simulink model "simTC"  (R2015a)
settings: Solver=ode4  StartTime=0.0  StopTime=T_sim  FixedStep=Ts  RelTol=1e-3
values from neighbouring files (symbols this model uses):
  A = [A, B; zeros(nu, nu+nx)]    [Main.m]    (also in longitudinal_inputRate.mat = [-0.0720238415998 -0.037172929775 0 2.59473518947e-15 0 0 8.; longitudinal_mat.mat = [-0.0720238415998 -0.037172929775 0 2.59473518947e-15 8.2339)
  B = [zeros(nx, nu); eye(nu)]    [Main.m]    (also in longitudinal_inputRate.mat = [0  0; 0  0; 0  0; 0  0; 1  0; 0  1]; longitudinal_mat.mat = [-0.11942228308  27.1604492573; -0.362246328988  0.037187163)
  C = [0 0 1 0 0 0]    [Main.m]    (also in main_CG.m = eye(nx); main_TC.m; main_TD.m = eye(nx))
  K_fb = K(:,1:nx)    [Main.m]    (also in main_TC.m)
  K_ff = K(:,nx+1:end)    [Main.m]    (also in main_TC.m)
  nx = size(Phi,1)    [CG_Offline.m]
  ref = 10    [Main.m]    (also in main_TC.m; main_TD.m)
undefined symbols (not defined in the file or in its folder): nu
settings Model: CovSFcnEnable=off  Creator=pier  LastModifiedBy=Piero
settings DebuggingCC: SolverPrmCheckMsg=warning

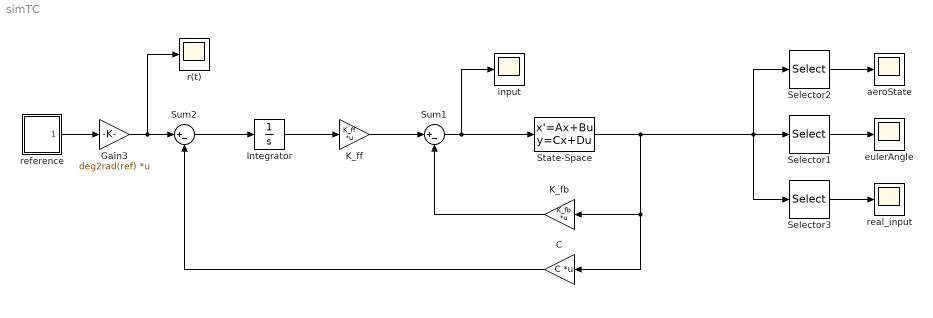
== system simTC ==
  C : Gain  Gain=C  Multiplication=Matrix(K*u)
  Gain3 : Gain  Gain=deg2rad(ref)  Multiplication=Matrix(K*u)
  Integrator : Integrator
  K_fb : Gain  Gain=K_fb  Multiplication=Matrix(K*u)
  K_ff : Gain  Gain=K_ff  Multiplication=Matrix(K*u)
  Selector1 : Selector  InputPortWidth=6  Indices=[3:4]
  Selector2 : Selector  InputPortWidth=6  Indices=[1:2]
  Selector3 : Selector  InputPortWidth=6  Indices=[5:6]
  State-Space : StateSpace  A=A  B=B  C=eye(nx)  D=zeros(nx,nu)  X0=0
  Sum1 : Sum  Inputs=|+-
  Sum2 : Sum  Inputs=|+-
  aeroState : Scope
      settings: TimeRange=100  SaveName=sim_aeroState
  eulerAngle : Scope
      settings: TimeRange=10  YMin=-0.025  YMax=0.275  SaveName=sim_eulerAngles
  input : Scope
      settings: TimeRange=20  SaveName=sim_Inputs
  r(t) : Scope
      settings: TimeRange=100  SaveName=sim_reference
  real_input : Scope
      settings: SaveName=sim_realInput  SampleInput=on  SampleTime=Ts
  reference : Subsystem
  wires:
  reference/1(Out1) -> Gain3/1
  Gain3/1 -> r(t)/1, Sum2/1
  Selector1/1 -> eulerAngle/1
  Selector3/1 -> real_input/1
  Selector2/1 -> aeroState/1
  State-Space/1 -> Selector3/1, Selector1/1, Selector2/1, K_fb/1, C/1
  Sum1/1 -> State-Space/1, input/1
  K_fb/1 -> Sum1/2
  C/1 -> Sum2/2
  Sum2/1 -> Integrator/1
  Integrator/1 -> K_ff/1
  K_ff/1 -> Sum1/1

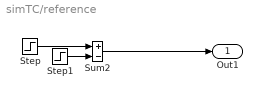
== system simTC/reference ==
  Step : Step  Time=2.5  SampleTime=0
  Step1 : Step  Time=12.5  SampleTime=0
  Sum2 : Sum  Inputs=+-
  Out1 : Outport
  wires:
  Sum2/1 -> Out1/1
  Step/1 -> Sum2/1
  Step1/1 -> Sum2/2
